simulink model "gm_fiter_model"  (R2021a)
settings: Solver=VariableStepAuto  StartTime=0.0  StopTime=10.0  RelTol=1e-3
libraries: hdlsllib x3
settings Model: Creator=MGMA  LastModifiedBy=MGMA
settings OptimizationCC: BlockReduction=off  ConditionallyExecuteInputs=off
settings DebuggingCC: InheritedTsInSrcMsg=none

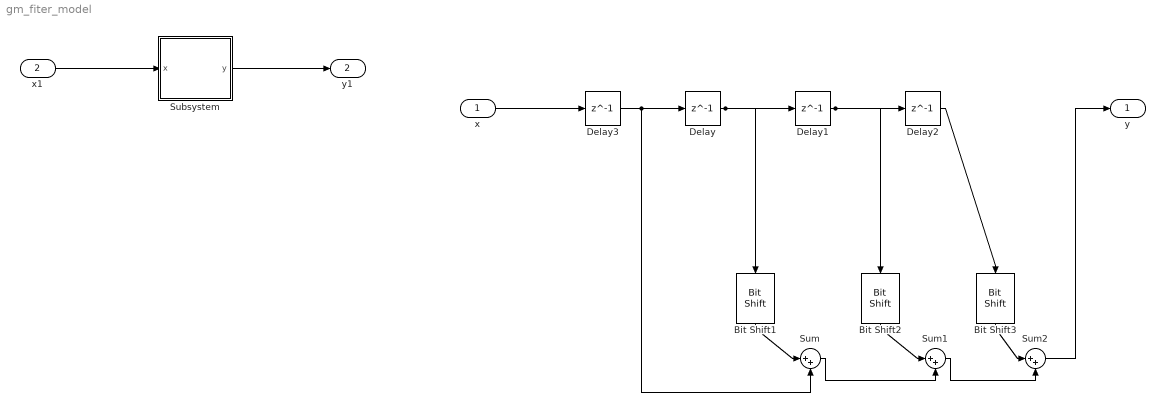
== system gm_fiter_model ==
  x : Inport  OutDataTypeStr=uint8  PortDimensions=1  SampleTime=0.2
  x1 : Inport  Port=2  OutDataTypeStr=uint8  PortDimensions=1  SampleTime=0.2
  Bit Shift1 : hdlsllib/Logic and Bit Operations/Bit Shift  mode=Shift Right Logical  N=1
  Bit Shift2 : hdlsllib/Logic and Bit Operations/Bit Shift  mode=Shift Right Logical  N=2
  Bit Shift3 : hdlsllib/Logic and Bit Operations/Bit Shift  mode=Shift Right Logical  N=3
  Delay{,1..3} (4 alike) : Delay  DelayLength=1  InitialCondition=0
  Subsystem : Subsystem
  Sum : Sum  Inputs=|++
  Sum1 : Sum  Inputs=|++
  Sum2 : Sum  Inputs=|++
  y : Outport  OutDataTypeStr=uint8  SampleTime=0.2
  y1 : Outport  Port=2  OutDataTypeStr=uint8  SampleTime=0.2
  wires:
  Bit Shift1/1 -> Sum/1
  Bit Shift2/1 -> Sum1/1
  Bit Shift3/1 -> Sum2/1
  Delay/1 -> Bit Shift1/1, Delay1/1
  Delay1/1 -> Bit Shift2/1, Delay2/1
  Delay2/1 -> Bit Shift3/1
  Sum/1 -> Sum1/2
  Sum1/1 -> Sum2/2
  Sum2/1 -> y/1
  Delay3/1 -> Sum/2, Delay/1
  x/1 -> Delay3/1
  x1/1 -> Subsystem/1(x)
  Subsystem/1(y) -> y1/1

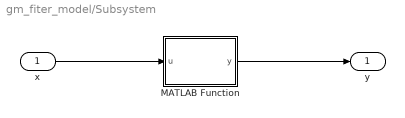
== system gm_fiter_model/Subsystem ==
  x : Inport  PortDimensions=1  SampleTime=0.2
  MATLAB Function : MATLAB Function  TreatAsAtomicUnit=on
  y : Outport  OutDataTypeStr=uint8  SampleTime=0.2
  wires:
  x/1 -> MATLAB Function/1(u)
  MATLAB Function/1(y) -> y/1

== matlab function gm_fiter_model/Subsystem/MATLAB Function ==
  data: u input; y output
function y = fcn(u)
H1 = 1;
H2 = 0.5;
H3 = 0.25;
H4 = 0.125;
x = u;     % Input signal
    % Shift delayed values
    delayed_x(4) = delayed_x(3);
    delayed_x(3) = delayed_x(2);
    delayed_x(2) = delayed_x(1);
    delayed_x(1) = x(i);
    % Compute the output
    y = unit8(floor(H1 * delayed_x(1)) + floor(H2 * delayed_x(2)) + floor(H3 * delayed_x(3)) + floor(H4 * delayed_x(4)));

end
